simulink model "observador_atualiza_so_quando_sensor"  (R2012b)
settings: Solver=ode3  StartTime=0.0  StopTime=10.0  FixedStep=1e-4  RelTol=1e-3
values from neighbouring files (symbols this model uses):
  A = [-0.2  0; 1  0]    [enc10_pulsegen0p5.mat]    (also in simulacaoBoaParaDebugar.mat)
  B = [10 0]    [enc10_pulsegen0p5.mat]    (also in simulacaoBoaParaDebugar.mat)
  C = [0 1]    [enc10_pulsegen0p5.mat]    (also in simulacaoBoaParaDebugar.mat)
libraries: Encoder x2, simulink x1
settings Model: Creator=Juliano  LastModifiedBy=Juliano

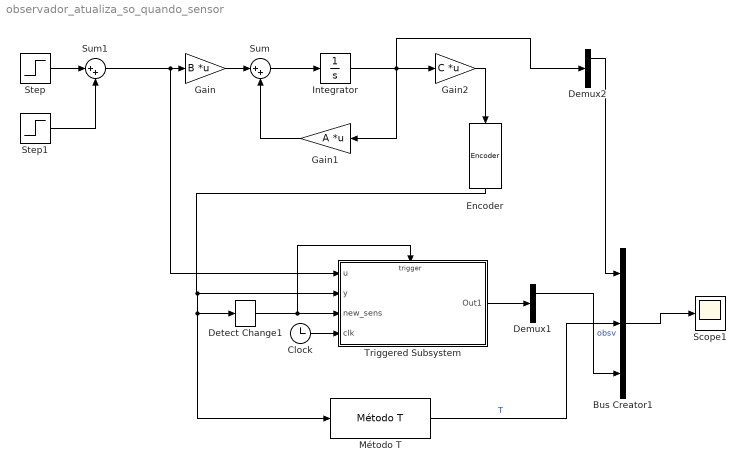
== system observador_atualiza_so_quando_sensor ==
  Bus Creator1 : BusCreator  Inputs=3
  Clock : Clock
  Demux1 : Demux  Outputs=2
  Demux2 : Demux  Outputs=2
  Detect Change1 : simulink/Logic and Bit Operations/Detect Change  vinit=0  InputProcessing=Inherited  OutDataTypeStr=boolean
  Encoder : Encoder/Encoder  Nr=10
  Gain : Gain  Gain=B  Multiplication=Matrix(K*u)
  Gain1 : Gain  Gain=A  Multiplication=Matrix(K*u)
  Gain2 : Gain  Gain=C  Multiplication=Matrix(K*u)
  Integrator : Integrator
  Método T : Encoder/Método T  m=1
  Scope1 : Scope
      settings: ShowLegends=on  TimeRange=10  YMin=-500  YMax=10000
  Step : Step  Time=0  After=20  SampleTime=0
  Step1 : Step  Time=5  After=-40  SampleTime=0
  Sum : Sum  Inputs=|++
  Sum1 : Sum  Inputs=|++
  Triggered Subsystem : Subsystem  TreatAsAtomicUnit=on
  wires:
  Gain/1 -> Sum/1
  Gain1/1 -> Sum/2
  Sum/1 -> Integrator/1
  Integrator/1 -> Gain1/1, Gain2/1, Demux2/1
  Step/1 -> Sum1/1
  Step1/1 -> Sum1/2
  Gain2/1 -> Encoder/1
  Sum1/1 -> Triggered Subsystem/1(u), Gain/1
  Clock/1 -> Triggered Subsystem/4(clk)
  Detect Change1/1 -> Triggered Subsystem/Trigger, Triggered Subsystem/3(new_sens)
  Encoder/1 -> Método T/1, Detect Change1/1, Triggered Subsystem/2(y)
  Triggered Subsystem/1(Out1) -> Demux1/1
  Demux2/1 -> Bus Creator1/1
  Demux1/1 -> Bus Creator1/3  "obsv"
  Método T/1 -> Bus Creator1/2  "T"
  Bus Creator1/1 -> Scope1/1

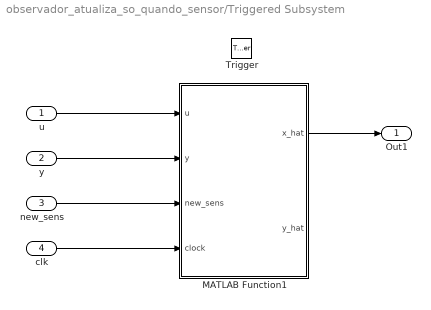
== system observador_atualiza_so_quando_sensor/Triggered Subsystem ==
  u : Inport
  y : Inport  Port=2
  new_sens : Inport  Port=3
  clk : Inport  Port=4
  Trigger : TriggerPort
  MATLAB Function1 : MATLAB Function  TreatAsAtomicUnit=on
  Out1 : Outport
  wires:
  new_sens/1 -> MATLAB Function1/3(new_sens)
  clk/1 -> MATLAB Function1/4(clock)
  y/1 -> MATLAB Function1/2(y)
  u/1 -> MATLAB Function1/1(u)
  MATLAB Function1/1(x_hat) -> Out1/1

== matlab function observador_atualiza_so_quando_sensor/Triggered Subsystem/MATLAB Function1 ==
  data: u input; y input; new_sens input; clock input; x_hat output; y_hat output
function [x_hat,y_hat] = fcn(u, y, new_sens, clock)

    %#codegen
    persistent x;
    persistent t;
    persistent C;
    persistent D;

    if(isempty(x) || isempty(t) || isempty(C) || isempty(D))
        x = [0 ; 0];
        t = 0;
        C = [0 1];
        D = 0;
    end

     if(new_sens == 1)
        deltaT = clock-t;
        A = [1-0.2*deltaT 0 ; deltaT 1];
        B = [10*deltaT; 0];
        L = [-0.18+0.2/deltaT+0.04*deltaT; 0.9-0.2*deltaT];
        x = A*x+B*u+L*(y-C*x);
     else
        deltaT = clock-t;
        A = [1-0.2*deltaT 0 ; deltaT 1];
        B = [10*deltaT; 0];
        x = A*x+B*u;
    end
    
    x_hat = x;
    y_hat = C*x+D*u;
    

    t = clock;
end
